simulink model "aperiodic"  (R2021b)
settings: Solver=VariableStepAuto  StartTime=0.0  StopTime=100.0  RelTol=1e-3
settings Model: Creator=iliya122  LastModifiedBy=Ivan
settings SolverCC: AlgebraicLoopSolver=TrustRegion
settings DebuggingCC: SFMachineParentedDataDiag=warning

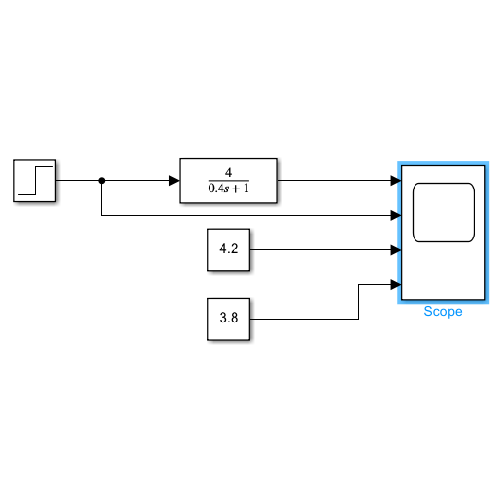
[thumbnail: Simulink's stored preview of the top-level diagram]
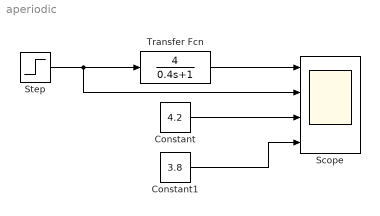
== system aperiodic ==
  Constant : Constant  Value=4.2
  Constant1 : Constant  Value=3.8
  Scope : Scope  NumInputPorts=4
  Step : Step  Time=2  SampleTime=0
  Transfer Fcn : TransferFcn  Numerator=4  Denominator=[0.4 1]
  wires:
  Step/1 -> Scope/2, Transfer Fcn/1
  Transfer Fcn/1 -> Scope/1
  Constant/1 -> Scope/3
  Constant1/1 -> Scope/4
